simulink model "SMC_03"  (R2021a)
settings: Solver=ode14x  StartTime=0.0  StopTime=100  FixedStep=0.01  RelTol=1e-3
libraries: simulink x2
settings Model: Creator=TMP  LastModifiedBy=TMP
settings DataIOCC: SaveTime=off  ReturnWorkspaceOutputs=off

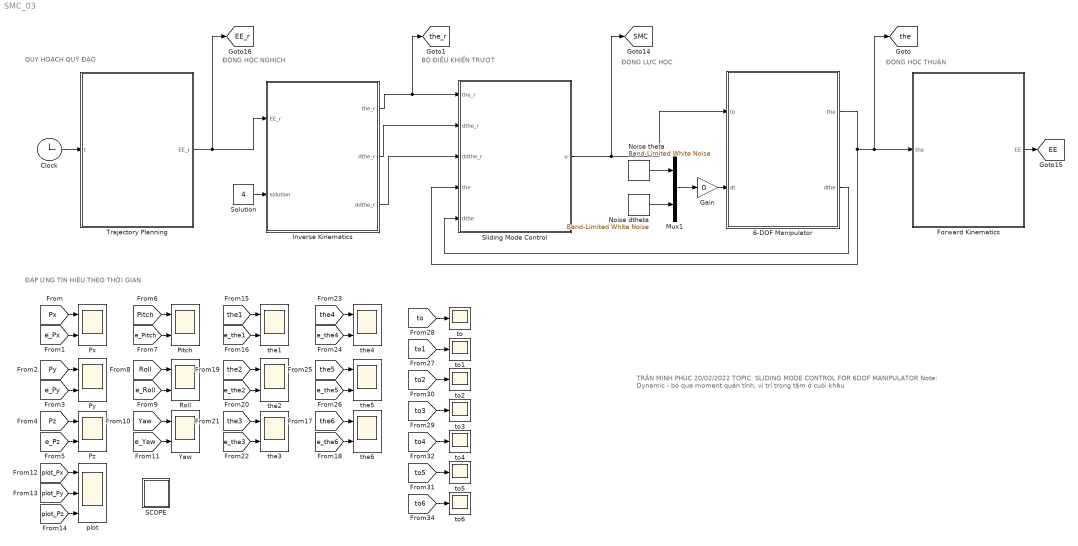
== system SMC_03 ==
  note: ĐÁP ỨNG TÍN HIÊU THEO THỜI GIAN
  note: QUY HOẠCH QUỸ ĐẠO
  note: BỘ ĐIỀU KHIỂN TRƯỢT
  note: ĐỘNG HỌC NGHỊCH
  note: ĐỌNG LỰC HỌC
  note: ĐỘNG HỌC THUẬN
  note: TRẦN MINH PHÚC
      | 20/02/2022
      | TOPIC: SLIDING MODE CONTROL FOR 6DOF MANIPULATOR
      | Note: Dynamic - bỏ qua moment quán tính, vị trí trọng tâm ở cuối khâu
  6-DOF Manipulator : Subsystem
  Clock : Clock
  Forward Kinematics : MATLAB Function  TreatAsAtomicUnit=on
  Gain : Gain  Gain=0
  Inverse Kinematics : Subsystem
  Mux1 : Mux  Inputs=2
  Noise dtheta : simulink/Sources/Band-Limited White Noise  Cov=[0.03]  Ts=0.01  seed=[23341]
  Noise theta : simulink/Sources/Band-Limited White Noise  Cov=[0.003]  Ts=0.01  seed=[23341]
  Pitch : Scope  NumInputPorts=2
  Px : Scope  NumInputPorts=2
  Py : Scope  NumInputPorts=2
  Pz : Scope  NumInputPorts=2
  Roll : Scope  NumInputPorts=2
  SCOPE : Subsystem
  Sliding Mode Control : MATLAB Function  TreatAsAtomicUnit=on
  Solution : Constant  Value=4
  Trajectory Planning : MATLAB Function  TreatAsAtomicUnit=on
  Yaw : Scope  NumInputPorts=2
  plot : Scope  NumInputPorts=3
  the{1..6} (6 alike) : Scope  NumInputPorts=2
  to{,1..6} (7 alike) : Scope
  tag scope: EE=global, EE_r=global, SMC=global, the=global, the_r=global
  wires:
  Noise theta/1 -> Mux1/1
  Noise dtheta/1 -> Mux1/2
  Mux1/1 -> Gain/1
  Clock/1 -> Trajectory Planning/1(t)
  Solution/1 -> Inverse Kinematics/2(solution)
  Trajectory Planning/1(EE_r) -> Inverse Kinematics/1(EE_r), [EE_r]
  [Px] -> Px/1
  [e_Px] -> Px/2
  [Py] -> Py/1
  [e_Py] -> Py/2
  [e_Pz] -> Pz/2
  [Pz] -> Pz/1
  [e_Yaw] -> Yaw/2
  [e_Roll] -> Roll/2
  [e_Pitch] -> Pitch/2
  [Yaw] -> Yaw/1
  [Roll] -> Roll/1
  [Pitch] -> Pitch/1
  [plot_Px] -> plot/1
  [plot_Py] -> plot/2
  [plot_Pz] -> plot/3
  [e_the5] -> the5/2
  [the5] -> the5/1
  [e_the4] -> the4/2
  [the4] -> the4/1
  [the3] -> the3/1
  [the2] -> the2/1
  [e_the6] -> the6/2
  [e_the2] -> the2/2
  [e_the1] -> the1/2
  [the6] -> the6/1
  [e_the3] -> the3/2
  [the1] -> the1/1
  [to1] -> to1/1
  [to] -> to/1
  [to6] -> to6/1
  [to5] -> to5/1
  [to4] -> to4/1
  [to3] -> to3/1
  [to2] -> to2/1
  Gain/1 -> 6-DOF Manipulator/2(dt)
  Sliding Mode Control/1(u) -> 6-DOF Manipulator/1(to), [SMC]
  6-DOF Manipulator/2(dthe) -> Sliding Mode Control/5(dthe)
  6-DOF Manipulator/1(the) -> Forward Kinematics/1(the), [the], Sliding Mode Control/4(the)
  Forward Kinematics/1(EE) -> [EE]
  Inverse Kinematics/1(the_r) -> [the_r], Sliding Mode Control/1(the_r)
  Inverse Kinematics/2(dthe_r) -> Sliding Mode Control/2(dthe_r)
  Inverse Kinematics/3(ddthe_r) -> Sliding Mode Control/3(ddthe_r)

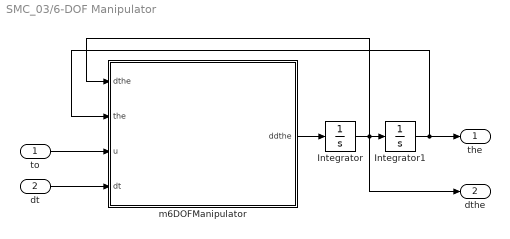
== system SMC_03/6-DOF Manipulator ==
  to : Inport
  dt : Inport  Port=2
  Integrator : Integrator  InitialCondition=[0.01;0.01;0.01;0.01;0.01;0.01]
  Integrator1 : Integrator  InitialCondition=[0.01;0.01;0.01;0.01;0.01;0.01]
  m6DOFManipulator : MATLAB Function  TreatAsAtomicUnit=on
  the : Outport
  dthe : Outport  Port=2
  wires:
  Integrator1/1 -> the/1, m6DOFManipulator/2(the)
  m6DOFManipulator/1(ddthe) -> Integrator/1
  Integrator/1 -> dthe/1, m6DOFManipulator/1(dthe), Integrator1/1
  dt/1 -> m6DOFManipulator/4(dt)
  to/1 -> m6DOFManipulator/3(u)

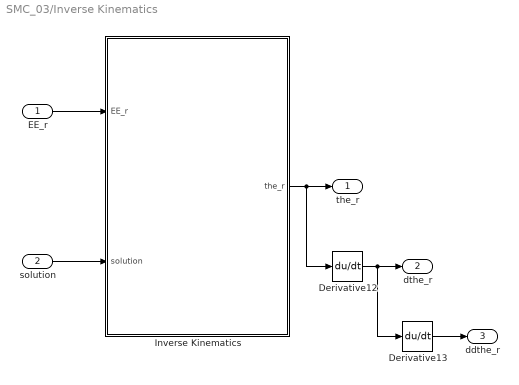
== system SMC_03/Inverse Kinematics ==
  EE_r : Inport
  solution : Inport  Port=2
  Derivative12 : Derivative
  Derivative13 : Derivative
  Inverse Kinematics : MATLAB Function  TreatAsAtomicUnit=on
  the_r : Outport  VectorParamsAs1DForOutWhenUnconnected=off
  dthe_r : Outport  Port=2  VectorParamsAs1DForOutWhenUnconnected=off
  ddthe_r : Outport  Port=3  VectorParamsAs1DForOutWhenUnconnected=off
  wires:
  EE_r/1 -> Inverse Kinematics/1(EE_r)
  solution/1 -> Inverse Kinematics/2(solution)
  Inverse Kinematics/1(the_r) -> Derivative12/1, the_r/1
  Derivative12/1 -> Derivative13/1, dthe_r/1
  Derivative13/1 -> ddthe_r/1

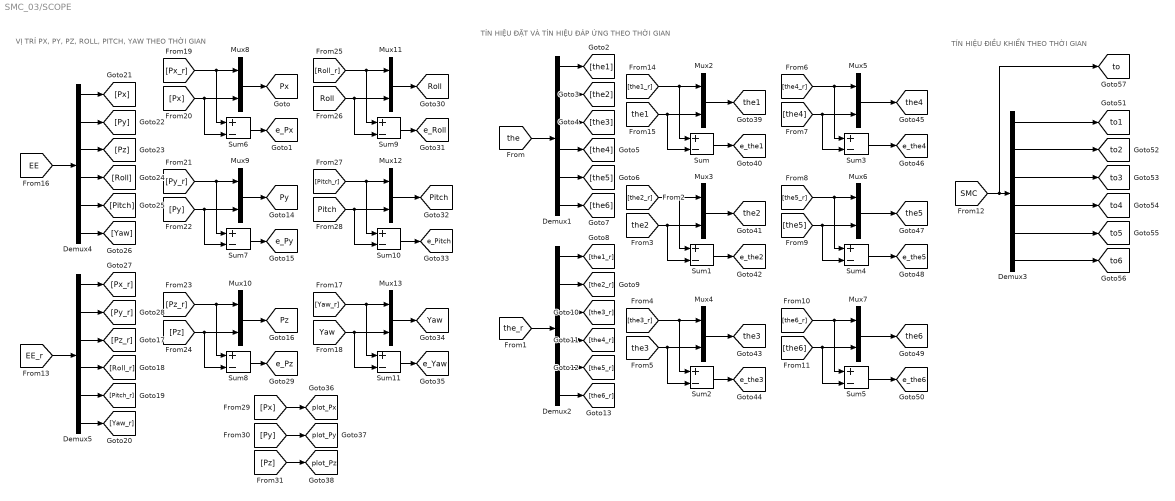
== system SMC_03/SCOPE ==
  note: TÍN HIỆU ĐIỀU KHIỂN THEO THỜI GIAN
  note: TÍN HIỆU ĐẶT VÀ TÍN HIỆU ĐÁP ỨNG THEO THỜI GIAN
  note: VỊ TRÍ PX, PY, PZ, ROLL, PITCH, YAW THEO THỜI GIAN
  Demux{1..5} (5 alike) : Demux  Outputs=6
  Mux{2..13} (12 alike) : Mux  Inputs=2
  Sum{,1..11} (12 alike) : Sum  Inputs=+-
  tag scope: Pitch=global, Px=global, Py=global, Pz=global, Roll=global, Yaw=global, e_Pitch=global, e_Px=global, e_Py=global, e_Pz=global, e_Roll=global, e_Yaw=global, e_the1=global, e_the2=global, e_the3=global, e_the4=global, e_the5=global, e_the6=global, plot_Px=global, plot_Py=global, plot_Pz=global, the1=global, the2=global, the3=global, the4=global, the5=global, the6=global, to1=global, to2=global, to3=global, to4=global, to5=global, to6=global, to=global
  wires:
  [the6] -> Sum5/2, Mux7/2
  Mux9/1 -> [Py]
  [the3] -> Sum2/2, Mux4/2
  Demux1/6 -> [the6]
  Demux5/1 -> [Px_r]
  [the1] -> Sum/2, Mux2/2
  [Py] -> Sum7/2, Mux9/2
  Demux2/2 -> [the2_r]
  Demux5/6 -> [Yaw_r]
  Demux4/4 -> [Roll]
  [Pz_r] -> Sum8/1, Mux10/1
  [the5] -> Sum4/2, Mux6/2
  [EE] -> Demux4/1
  Mux11/1 -> [Roll]
  [EE_r] -> Demux5/1
  Demux4/2 -> [Py]
  [Px_r] -> Sum6/1, Mux8/1
  Mux5/1 -> [the4]
  Demux1/4 -> [the4]
  [Pitch] -> Sum10/2, Mux12/2
  [the6_r] -> Sum5/1, Mux7/1
  Mux2/1 -> [the1]
  [the4_r] -> Sum3/1, Mux5/1
  Demux2/1 -> [the1_r]
  Demux5/5 -> [Pitch_r]
  [the1_r] -> Sum/1, Mux2/1
  Sum7/1 -> [e_Py]
  Demux4/3 -> [Pz]
  [Py_r] -> Sum7/1, Mux9/1
  Demux1/3 -> [the3]
  Demux5/2 -> [Py_r]
  Demux3/1 -> [to1]
  Demux4/6 -> [Yaw]
  [Pz] -> [plot_Pz]
  [Roll] -> Sum9/2, Mux11/2
  Demux5/3 -> [Pz_r]
  [Roll_r] -> Sum9/1, Mux11/1
  Demux2/5 -> [the5_r]
  [Px] -> Sum6/2, Mux8/2
  [the5_r] -> Sum4/1, Mux6/1
  Demux5/4 -> [Roll_r]
  [the] -> Demux1/1
  Demux1/2 -> [the2]
  Demux1/1 -> [the1]
  Mux7/1 -> [the6]
  Demux2/4 -> [the4_r]
  [Yaw_r] -> Sum11/1, Mux13/1
  [the_r] -> Demux2/1
  Demux3/3 -> [to3]
  [the2_r] -> Sum1/1, Mux3/1
  Demux4/1 -> [Px]
  [Pitch_r] -> Sum10/1, Mux12/1
  [Pz] -> Sum8/2, Mux10/2
  Demux2/6 -> [the6_r]
  [SMC] -> [to], Demux3/1
  Sum9/1 -> [e_Roll]
  [the3_r] -> Sum2/1, Mux4/1
  [Yaw] -> Sum11/2, Mux13/2
  Sum8/1 -> [e_Pz]
  Demux2/3 -> [the3_r]
  Demux1/5 -> [the5]
  [the4] -> Sum3/2, Mux5/2
  [the2] -> Sum1/2, Mux3/2
  Demux4/5 -> [Pitch]
  Sum11/1 -> [e_Yaw]
  [Px] -> [plot_Px]
  Sum6/1 -> [e_Px]
  [Py] -> [plot_Py]
  Mux3/1 -> [the2]
  Sum/1 -> [e_the1]
  Sum5/1 -> [e_the6]
  Sum2/1 -> [e_the3]
  Sum4/1 -> [e_the5]
  Mux4/1 -> [the3]
  Sum1/1 -> [e_the2]
  Demux3/4 -> [to4]
  Mux6/1 -> [the5]
  Demux3/5 -> [to5]
  Mux13/1 -> [Yaw]
  Sum3/1 -> [e_the4]
  Demux3/6 -> [to6]
  Mux10/1 -> [Pz]
  Mux8/1 -> [Px]
  Demux3/2 -> [to2]
  Mux12/1 -> [Pitch]
  Sum10/1 -> [e_Pitch]

== matlab function SMC_03/Sliding Mode Control ==
  data: the_r input; dthe_r input; ddthe_r input; the input; u output; dthe input
function u = SMC(the_r,dthe_r,ddthe_r,the,dthe)
%% Declare manipulator dynamics:
m1=0.1; m2=0.1; m3=0.1; m4=0.1; m5=0.1; m6=0.1;
I1=0; I2=0; I3=0; I4=0; I5=0; I6=1;
a1=0.75; a2=2.70; a3=0.90; d1=3.35; d4=2.95; d7=0.80;
g=9.81;
%%
e1 = the(1); e2 = the(2); e3 = the(3);
e4 = the(4); e5 = the(5); e6 = the(6);
de1 = dthe(1); de2 = dthe(2); de3 = dthe(3);
de4 = dthe(4); de5 = dthe(5); de6 = dthe(6);
%% M
M = [I1 + I2 + I3 + I4 + I5 + I6 + a1^2*m2 + a1^2*m3 + a1^2*m4 + (a2^2*m3)/2 + a1^2*m5 + (a2^2*m4)/2 + a1^2*m6 + (a2^2*m5)/2 + (a3^2*m4)/2 + (a2^2*m6)/2 + (a3^2*m5)/2 + (a3^2*m6)/2 + (d4^2*m4)/2 + (d4^2*m5)/2 + (d4^2*m6)/2 - (a2^2*m3*cos(2*e2))/2 - (a2^2*m4*cos(2*e2))/2 - (a2^2*m5*cos(2*e2))/2 - (a2^2*m6*cos(2*e2))/2 - (a3^2*m4*cos(2*e2 + 2*e3))/2 - (a3^2*m5*cos(2*e2 + 2*e3))/2 - (a3^2*m6*cos(2*e2 + 2*e3))/2 + (d4^2*m4*cos(2*e2 + 2*e3))/2 + (d4^2*m5*cos(2*e2 + 2*e3))/2 + (d4^2*m6*cos(2*e2 + 2*e3))/2 + 2*a1*d4*m4*cos(e2 + e3) + 2*a1*d4*m5*cos(e2 + e3) + 2*a1*d4*m6*cos(e2 + e3) + 2*a1*a3*m4*sin(e2 + e3) + 2*a1*a3*m5*sin(e2 + e3) + 2*a1*a3*m6*sin(e2 + e3) + a2*a3*m4*cos(e3) + a2*a3*m5*cos(e3) + a2*a3*m6*cos(e3) + 2*a1*a2*m3*sin(e2) + 2*a1*a2*m4*sin(e2) + 2*a1*a2*m5*sin(e2) + 2*a1*a2*m6*sin(e2) - a2*d4*m4*sin(e3) - a2*d4*m5*sin(e3) - a2*d4*m6*sin(e3) - a2*a3*m4*cos(2*e2 + e3) - a2*a3*m5*cos(2*e2 + e3) - a2*a3*m6*cos(2*e2 + e3) + a2*d4*m4*sin(2*e2 + e3) + a2*d4*m5*sin(2*e2 + e3) + a2*d4*m6*sin(2*e2 + e3) + a3*d4*m4*sin(2*e2 + 2*e3) + a3*d4*m5*sin(2*e2 + 2*e3) + a3*d4*m6*sin(2*e2 + 2*e3),0,0,-sin(e2 + e3)*(I4 + I5 + I6),cos(e2 + e3)*sin(e4)*(I5 + I6),I6*cos(e4)*sin(e2)*sin(e3)*sin(e5) - I6*cos(e3)*cos(e5)*sin(e2) - I6*cos(e2)*cos(e3)*cos(e4)*sin(e5) - I6*cos(e2)*cos(e5)*sin(e3);
     0,I2 + I3 + I4 + I5 + I6 + a2^2*m3 + a2^2*m4 + a2^2*m5 + a3^2*m4 + a2^2*m6 + a3^2*m5 + a3^2*m6 + d4^2*m4 + d4^2*m5 + d4^2*m6 + 2*a2*a3*m4*cos(e3) + 2*a2*a3*m5*cos(e3) + 2*a2*a3*m6*cos(e3) - 2*a2*d4*m4*sin(e3) - 2*a2*d4*m5*sin(e3) - 2*a2*d4*m6*sin(e3),I3 + I4 + I5 + I6 + a3^2*m4 + a3^2*m5 + a3^2*m6 + d4^2*m4 + d4^2*m5 + d4^2*m6 + a2*a3*m4*cos(e3) + a2*a3*m5*cos(e3) + a2*a3*m6*cos(e3) - a2*d4*m4*sin(e3) - a2*d4*m5*sin(e3) - a2*d4*m6*sin(e3),0,cos(e4)*(I5 + I6),I6*sin(e4)*sin(e5);
     0,I3 + I4 + I5 + I6 + a3^2*m4 + a3^2*m5 + a3^2*m6 + d4^2*m4 + d4^2*m5 + d4^2*m6 + a2*a3*m4*cos(e3) + a2*a3*m5*cos(e3) + a2*a3*m6*cos(e3) - a2*d4*m4*sin(e3) - a2*d4*m5*sin(e3) - a2*d4*m6*sin(e3),I3 + I4 + I5 + I6 + a3^2*m4 + a3^2*m5 + a3^2*m6 + d4^2*m4 + d4^2*m5 + d4^2*m6,0,cos(e4)*(I5 + I6),I6*sin(e4)*sin(e5);
    -sin(e2 + e3)*(I4 + I5 + I6),0,0,I4 + I5 + I6,0,I6*cos(e5);
    cos(e2 + e3)*sin(e4)*(I5 + I6),cos(e4)*(I5 + I6),cos(e4)*(I5 + I6),0,I5 + I6,0;
    I6*cos(e4)*sin(e2)*sin(e3)*sin(e5) - I6*cos(e3)*cos(e5)*sin(e2) - I6*cos(e2)*cos(e3)*cos(e4)*sin(e5) - I6*cos(e2)*cos(e5)*sin(e3),I6*sin(e4)*sin(e5),I6*sin(e4)*sin(e5),I6*cos(e5),0,I6];
%% C
C = ...
[de2*(a2^2*m3*sin(2*e2) + a2^2*m4*sin(2*e2) + a2^2*m5*sin(2*e2) + a2^2*m6*sin(2*e2) + a3^2*m4*sin(2*e2 + 2*e3) + a3^2*m5*sin(2*e2 + 2*e3) + a3^2*m6*sin(2*e2 + 2*e3) - d4^2*m4*sin(2*e2 + 2*e3) - d4^2*m5*sin(2*e2 + 2*e3) - d4^2*m6*sin(2*e2 + 2*e3) + 2*a1*a3*m4*cos(e2 + e3) + 2*a1*a3*m5*cos(e2 + e3) + 2*a1*a3*m6*cos(e2 + e3) - 2*a1*d4*m4*sin(e2 + e3) - 2*a1*d4*m5*sin(e2 + e3) - 2*a1*d4*m6*sin(e2 + e3) + 2*a1*a2*m3*cos(e2) + 2*a1*a2*m4*cos(e2) + 2*a1*a2*m5*cos(e2) + 2*a1*a2*m6*cos(e2) + 2*a2*d4*m4*cos(2*e2 + e3) + 2*a2*d4*m5*cos(2*e2 + e3) + 2*a2*d4*m6*cos(2*e2 + e3) + 2*a2*a3*m4*sin(2*e2 + e3) + 2*a2*a3*m5*sin(2*e2 + e3) + 2*a2*a3*m6*sin(2*e2 + e3) + 2*a3*d4*m4*cos(2*e2 + 2*e3) + 2*a3*d4*m5*cos(2*e2 + 2*e3) + 2*a3*d4*m6*cos(2*e2 + 2*e3)) + de3*(m4 + m5 + m6)*(a3^2*sin(2*e2 + 2*e3) - d4^2*sin(2*e2 + 2*e3) + a2*d4*cos(2*e2 + e3) + a2*a3*sin(2*e2 + e3) + 2*a3*d4*cos(2*e2 + 2*e3) + 2*a1*a3*cos(e2 + e3) - 2*a1*d4*sin(e2 + e3) - a2*d4*cos(e3) - a2*a3*sin(e3)),0,0,-cos(e2 + e3)*(de2 + de3)*(I4 + I5 + I6),-(I5 + I6)*(de2*sin(e2 + e3)*sin(e4) - de4*cos(e2 + e3)*cos(e4) + de3*sin(e2 + e3)*sin(e4)),I6*de2*(cos(e5)*sin(e2)*sin(e3) - cos(e2)*cos(e3)*cos(e5) + cos(e2)*cos(e4)*sin(e3)*sin(e5) + cos(e3)*cos(e4)*sin(e2)*sin(e5)) + I6*de3*(cos(e5)*sin(e2)*sin(e3) - cos(e2)*cos(e3)*cos(e5) + cos(e2)*cos(e4)*sin(e3)*sin(e5) + cos(e3)*cos(e4)*sin(e2)*sin(e5)) + I6*de5*(cos(e2)*sin(e3)*sin(e5) + cos(e3)*sin(e2)*sin(e5) - cos(e2)*cos(e3)*cos(e4)*cos(e5) + cos(e4)*cos(e5)*sin(e2)*sin(e3)) + I6*de4*cos(e2 + e3)*sin(e4)*sin(e5);
 (I4*de4*cos(e2 + e3))/2 + (I5*de4*cos(e2 + e3))/2 + (I6*de4*cos(e2 + e3))/2 - (a2^2*de1*m3*sin(2*e2))/2 - (a2^2*de1*m4*sin(2*e2))/2 - (a2^2*de1*m5*sin(2*e2))/2 - (a2^2*de1*m6*sin(2*e2))/2 - (a3^2*de1*m4*sin(2*e2 + 2*e3))/2 - (a3^2*de1*m5*sin(2*e2 + 2*e3))/2 - (a3^2*de1*m6*sin(2*e2 + 2*e3))/2 + (d4^2*de1*m4*sin(2*e2 + 2*e3))/2 + (d4^2*de1*m5*sin(2*e2 + 2*e3))/2 + (d4^2*de1*m6*sin(2*e2 + 2*e3))/2 + (I5*de5*sin(e2 + e3)*sin(e4))/2 + (I6*de5*sin(e2 + e3)*sin(e4))/2 - a3*d4*de1*m4*cos(2*e2 + 2*e3) - a3*d4*de1*m5*cos(2*e2 + 2*e3) - a3*d4*de1*m6*cos(2*e2 + 2*e3) + (I6*de6*cos(e2)*cos(e3)*cos(e5))/2 - a1*a3*de1*m4*cos(e2 + e3) - a1*a3*de1*m5*cos(e2 + e3) - a1*a3*de1*m6*cos(e2 + e3) - (I6*de6*cos(e5)*sin(e2)*sin(e3))/2 + a1*d4*de1*m4*sin(e2 + e3) + a1*d4*de1*m5*sin(e2 + e3) + a1*d4*de1*m6*sin(e2 + e3) - a1*a2*de1*m3*cos(e2) - a1*a2*de1*m4*cos(e2) - a1*a2*de1*m5*cos(e2) - a1*a2*de1*m6*cos(e2) - a2*d4*de1*m4*cos(2*e2 + e3) - a2*d4*de1*m5*cos(2*e2 + e3) - a2*d4*de1*m6*cos(2*e2 + e3) - a2*a3*de1*m4*sin(2*e2 + e3) - a2*a3*de1*m5*sin(2*e2 + e3) - a2*a3*de1*m6*sin(2*e2 + e3) - (I6*de6*cos(e2)*cos(e4)*sin(e3)*sin(e5))/2 - (I6*de6*cos(e3)*cos(e4)*sin(e2)*sin(e5))/2,-2*a2*de3*(d4*cos(e3) + a3*sin(e3))*(m4 + m5 + m6),-a2*de3*(d4*cos(e3) + a3*sin(e3))*(m4 + m5 + m6),(de1*cos(e2 + e3)*(I4 + I5 + I6))/2,-(sin(e4)*(2*de4 - de1*sin(e2 + e3))*(I5 + I6))/2,(I6*(2*de4*cos(e4)*sin(e5) + 2*de5*cos(e5)*sin(e4) + de1*cos(e2)*cos(e3)*cos(e5) - de1*cos(e5)*sin(e2)*sin(e3) - de1*cos(e2)*cos(e4)*sin(e3)*sin(e5) - de1*cos(e3)*cos(e4)*sin(e2)*sin(e5)))/2;
 (de4*cos(e2 + e3)*(I4 + I5 + I6))/2 - (I6*de6*(cos(e5)*sin(e2)*sin(e3) - cos(e2)*cos(e3)*cos(e5) + cos(e2)*cos(e4)*sin(e3)*sin(e5) + cos(e3)*cos(e4)*sin(e2)*sin(e5)))/2 - (de1*(m4 + m5 + m6)*(a3^2*sin(2*e2 + 2*e3) - d4^2*sin(2*e2 + 2*e3) + a2*d4*cos(2*e2 + e3) + a2*a3*sin(2*e2 + e3) + 2*a3*d4*cos(2*e2 + 2*e3) + 2*a1*a3*cos(e2 + e3) - 2*a1*d4*sin(e2 + e3) - a2*d4*cos(e3) - a2*a3*sin(e3)))/2 + (de5*sin(e2 + e3)*sin(e4)*(I5 + I6))/2,(a2*(d4*cos(e3) + a3*sin(e3))*(2*de2 - de3)*(m4 + m5 + m6))/2,(a2*de2*(d4*cos(e3) + a3*sin(e3))*(m4 + m5 + m6))/2,(de1*cos(e2 + e3)*(I4 + I5 + I6))/2,-(sin(e4)*(2*de4 - de1*sin(e2 + e3))*(I5 + I6))/2,(I6*(2*de4*cos(e4)*sin(e5) + 2*de5*cos(e5)*sin(e4) + de1*cos(e2)*cos(e3)*cos(e5) - de1*cos(e5)*sin(e2)*sin(e3) - de1*cos(e2)*cos(e4)*sin(e3)*sin(e5) - de1*cos(e3)*cos(e4)*sin(e2)*sin(e5)))/2;
 - cos(e2 + e3)*(de2 + de3)*(I4 + I5 + I6) - (de5*cos(e2 + e3)*cos(e4)*(I5 + I6))/2 - (I6*de6*cos(e2 + e3)*sin(e4)*sin(e5))/2,(de5*sin(e4)*(I5 + I6))/2 - (I6*de6*cos(e4)*sin(e5))/2,(de5*sin(e4)*(I5 + I6))/2 - (I6*de6*cos(e4)*sin(e5))/2,0,((I5 + I6)*(de2*sin(e4) + de3*sin(e4) - de1*cos(e2 + e3)*cos(e4)))/2,-(I6*sin(e5)*(2*de5 + de2*cos(e4) + de3*cos(e4) + de1*cos(e2 + e3)*sin(e4)))/2;
 - (I5 + I6)*(de2*sin(e2 + e3)*sin(e4) - de4*cos(e2 + e3)*cos(e4) + de3*sin(e2 + e3)*sin(e4)) - (I6*de6*(cos(e2)*sin(e3)*sin(e5) + cos(e3)*sin(e2)*sin(e5) - cos(e2)*cos(e3)*cos(e4)*cos(e5) + cos(e4)*cos(e5)*sin(e2)*sin(e3)))/2,- de4*sin(e4)*(I5 + I6) - (I6*de6*cos(e5)*sin(e4))/2,- de4*sin(e4)*(I5 + I6) - (I6*de6*cos(e5)*sin(e4))/2,(I6*de6*sin(e5))/2,0,-(I6*(de2*cos(e5)*sin(e4) - de4*sin(e5) + de3*cos(e5)*sin(e4) + de1*cos(e2)*sin(e3)*sin(e5) + de1*cos(e3)*sin(e2)*sin(e5) + de1*cos(e4)*cos(e5)*sin(e2)*sin(e3) - de1*cos(e2)*cos(e3)*cos(e4)*cos(e5)))/2;
 I6*de2*(cos(e5)*sin(e2)*sin(e3) - cos(e2)*cos(e3)*cos(e5) + cos(e2)*cos(e4)*sin(e3)*sin(e5) + cos(e3)*cos(e4)*sin(e2)*sin(e5)) + I6*de3*(cos(e5)*sin(e2)*sin(e3) - cos(e2)*cos(e3)*cos(e5) + cos(e2)*cos(e4)*sin(e3)*sin(e5) + cos(e3)*cos(e4)*sin(e2)*sin(e5)) + I6*de5*(cos(e2)*sin(e3)*sin(e5) + cos(e3)*sin(e2)*sin(e5) - cos(e2)*cos(e3)*cos(e4)*cos(e5) + cos(e4)*cos(e5)*sin(e2)*sin(e3)) + I6*de4*cos(e2 + e3)*sin(e4)*sin(e5),I6*de4*cos(e4)*sin(e5) + I6*de5*cos(e5)*sin(e4),I6*de4*cos(e4)*sin(e5) + I6*de5*cos(e5)*sin(e4),-I6*de5*sin(e5),0,0];
%% V
V = C*dthe;
%% G
G = ...
[    
                                                                                                                                                                                              0;
g*(a2*m3*sin(e2) + a2*m4*sin(e2) + a2*m5*sin(e2) + a2*m6*sin(e2) + d4*m4*cos(e2 + e3) + d4*m5*cos(e2 + e3) + d4*m6*cos(e2 + e3) + a3*m4*sin(e2 + e3) + a3*m5*sin(e2 + e3) + a3*m6*sin(e2 + e3));
                                                                                                                                           g*(d4*cos(e2 + e3) + a3*sin(e2 + e3))*(m4 + m5 + m6);
                                                                                                                                                                                              0;
                                                                                                                                                                                              0;
                                                                                                                                                                                              0];

%% Control:
% Controler parameters
% % with noise
% lamda = 50;
% K = 30;
% K1 = 50;

% without noise
lamda = diag([20,20,20,20,20,20]);
K = diag([20,20,20,20,20,20]);
K1 = diag([5,5,5,5,5,5]);

% Designed sliding mode control
f_x = -inv(M)*V - inv(M)*G;
g_x = inv(M);
e1 = the - the_r;
e2 = dthe - dthe_r;
s = lamda*e1 + e2;
u = inv(g_x)*(-f_x + ddthe_r - lamda*e2 - K1*s - K*sign(s));
% sat
% u = inv(g_x)*(-f_x + ddthe_r - lamda*e2 - K1*s - K*min(0.1, max(-0.1, s)));

== matlab function SMC_03/6-DOF Manipulator/m6DOFManipulator ==
  data: dthe input; the input; u input; ddthe output; dt input
function ddthe  = m6DOFManipulator(dthe,the,u,dt)
%% Declare:
m1=0.1; m2=0.1; m3=0.1; m4=0.1; m5=0.1; m6=0.1;
I1=0; I2=0; I3=0; I4=0; I5=0; I6=1;
a1=0.75; a2=2.70; a3=0.90; d1=3.35; d4=2.95; d7=0.80;
g=9.81;
%%
e1 = the(1) + dt(1); e2 = the(2) + dt(1); e3 = the(3) + dt(1);
e4 = the(4) + dt(1); e5 = the(5) + dt(1); e6 = the(6) + dt(1);
de1 = dthe(1) + dt(2); de2 = dthe(2) + dt(2); de3 = dthe(3) + dt(2);
de4 = dthe(4) + dt(2); de5 = dthe(5) + dt(2); de6 = dthe(6) + dt(2);
%% M
M = [I1 + I2 + I3 + I4 + I5 + I6 + a1^2*m2 + a1^2*m3 + a1^2*m4 + (a2^2*m3)/2 + a1^2*m5 + (a2^2*m4)/2 + a1^2*m6 + (a2^2*m5)/2 + (a3^2*m4)/2 + (a2^2*m6)/2 + (a3^2*m5)/2 + (a3^2*m6)/2 + (d4^2*m4)/2 + (d4^2*m5)/2 + (d4^2*m6)/2 - (a2^2*m3*cos(2*e2))/2 - (a2^2*m4*cos(2*e2))/2 - (a2^2*m5*cos(2*e2))/2 - (a2^2*m6*cos(2*e2))/2 - (a3^2*m4*cos(2*e2 + 2*e3))/2 - (a3^2*m5*cos(2*e2 + 2*e3))/2 - (a3^2*m6*cos(2*e2 + 2*e3))/2 + (d4^2*m4*cos(2*e2 + 2*e3))/2 + (d4^2*m5*cos(2*e2 + 2*e3))/2 + (d4^2*m6*cos(2*e2 + 2*e3))/2 + 2*a1*d4*m4*cos(e2 + e3) + 2*a1*d4*m5*cos(e2 + e3) + 2*a1*d4*m6*cos(e2 + e3) + 2*a1*a3*m4*sin(e2 + e3) + 2*a1*a3*m5*sin(e2 + e3) + 2*a1*a3*m6*sin(e2 + e3) + a2*a3*m4*cos(e3) + a2*a3*m5*cos(e3) + a2*a3*m6*cos(e3) + 2*a1*a2*m3*sin(e2) + 2*a1*a2*m4*sin(e2) + 2*a1*a2*m5*sin(e2) + 2*a1*a2*m6*sin(e2) - a2*d4*m4*sin(e3) - a2*d4*m5*sin(e3) - a2*d4*m6*sin(e3) - a2*a3*m4*cos(2*e2 + e3) - a2*a3*m5*cos(2*e2 + e3) - a2*a3*m6*cos(2*e2 + e3) + a2*d4*m4*sin(2*e2 + e3) + a2*d4*m5*sin(2*e2 + e3) + a2*d4*m6*sin(2*e2 + e3) + a3*d4*m4*sin(2*e2 + 2*e3) + a3*d4*m5*sin(2*e2 + 2*e3) + a3*d4*m6*sin(2*e2 + 2*e3),0,0,-sin(e2 + e3)*(I4 + I5 + I6),cos(e2 + e3)*sin(e4)*(I5 + I6),I6*cos(e4)*sin(e2)*sin(e3)*sin(e5) - I6*cos(e3)*cos(e5)*sin(e2) - I6*cos(e2)*cos(e3)*cos(e4)*sin(e5) - I6*cos(e2)*cos(e5)*sin(e3);
     0,I2 + I3 + I4 + I5 + I6 + a2^2*m3 + a2^2*m4 + a2^2*m5 + a3^2*m4 + a2^2*m6 + a3^2*m5 + a3^2*m6 + d4^2*m4 + d4^2*m5 + d4^2*m6 + 2*a2*a3*m4*cos(e3) + 2*a2*a3*m5*cos(e3) + 2*a2*a3*m6*cos(e3) - 2*a2*d4*m4*sin(e3) - 2*a2*d4*m5*sin(e3) - 2*a2*d4*m6*sin(e3),I3 + I4 + I5 + I6 + a3^2*m4 + a3^2*m5 + a3^2*m6 + d4^2*m4 + d4^2*m5 + d4^2*m6 + a2*a3*m4*cos(e3) + a2*a3*m5*cos(e3) + a2*a3*m6*cos(e3) - a2*d4*m4*sin(e3) - a2*d4*m5*sin(e3) - a2*d4*m6*sin(e3),0,cos(e4)*(I5 + I6),I6*sin(e4)*sin(e5);
     0,I3 + I4 + I5 + I6 + a3^2*m4 + a3^2*m5 + a3^2*m6 + d4^2*m4 + d4^2*m5 + d4^2*m6 + a2*a3*m4*cos(e3) + a2*a3*m5*cos(e3) + a2*a3*m6*cos(e3) - a2*d4*m4*sin(e3) - a2*d4*m5*sin(e3) - a2*d4*m6*sin(e3),I3 + I4 + I5 + I6 + a3^2*m4 + a3^2*m5 + a3^2*m6 + d4^2*m4 + d4^2*m5 + d4^2*m6,0,cos(e4)*(I5 + I6),I6*sin(e4)*sin(e5);
    -sin(e2 + e3)*(I4 + I5 + I6),0,0,I4 + I5 + I6,0,I6*cos(e5);
    cos(e2 + e3)*sin(e4)*(I5 + I6),cos(e4)*(I5 + I6),cos(e4)*(I5 + I6),0,I5 + I6,0;
    I6*cos(e4)*sin(e2)*sin(e3)*sin(e5) - I6*cos(e3)*cos(e5)*sin(e2) - I6*cos(e2)*cos(e3)*cos(e4)*sin(e5) - I6*cos(e2)*cos(e5)*sin(e3),I6*sin(e4)*sin(e5),I6*sin(e4)*sin(e5),I6*cos(e5),0,I6];
%% C
C = ...
[de2*(a2^2*m3*sin(2*e2) + a2^2*m4*sin(2*e2) + a2^2*m5*sin(2*e2) + a2^2*m6*sin(2*e2) + a3^2*m4*sin(2*e2 + 2*e3) + a3^2*m5*sin(2*e2 + 2*e3) + a3^2*m6*sin(2*e2 + 2*e3) - d4^2*m4*sin(2*e2 + 2*e3) - d4^2*m5*sin(2*e2 + 2*e3) - d4^2*m6*sin(2*e2 + 2*e3) + 2*a1*a3*m4*cos(e2 + e3) + 2*a1*a3*m5*cos(e2 + e3) + 2*a1*a3*m6*cos(e2 + e3) - 2*a1*d4*m4*sin(e2 + e3) - 2*a1*d4*m5*sin(e2 + e3) - 2*a1*d4*m6*sin(e2 + e3) + 2*a1*a2*m3*cos(e2) + 2*a1*a2*m4*cos(e2) + 2*a1*a2*m5*cos(e2) + 2*a1*a2*m6*cos(e2) + 2*a2*d4*m4*cos(2*e2 + e3) + 2*a2*d4*m5*cos(2*e2 + e3) + 2*a2*d4*m6*cos(2*e2 + e3) + 2*a2*a3*m4*sin(2*e2 + e3) + 2*a2*a3*m5*sin(2*e2 + e3) + 2*a2*a3*m6*sin(2*e2 + e3) + 2*a3*d4*m4*cos(2*e2 + 2*e3) + 2*a3*d4*m5*cos(2*e2 + 2*e3) + 2*a3*d4*m6*cos(2*e2 + 2*e3)) + de3*(m4 + m5 + m6)*(a3^2*sin(2*e2 + 2*e3) - d4^2*sin(2*e2 + 2*e3) + a2*d4*cos(2*e2 + e3) + a2*a3*sin(2*e2 + e3) + 2*a3*d4*cos(2*e2 + 2*e3) + 2*a1*a3*cos(e2 + e3) - 2*a1*d4*sin(e2 + e3) - a2*d4*cos(e3) - a2*a3*sin(e3)),0,0,-cos(e2 + e3)*(de2 + de3)*(I4 + I5 + I6),-(I5 + I6)*(de2*sin(e2 + e3)*sin(e4) - de4*cos(e2 + e3)*cos(e4) + de3*sin(e2 + e3)*sin(e4)),I6*de2*(cos(e5)*sin(e2)*sin(e3) - cos(e2)*cos(e3)*cos(e5) + cos(e2)*cos(e4)*sin(e3)*sin(e5) + cos(e3)*cos(e4)*sin(e2)*sin(e5)) + I6*de3*(cos(e5)*sin(e2)*sin(e3) - cos(e2)*cos(e3)*cos(e5) + cos(e2)*cos(e4)*sin(e3)*sin(e5) + cos(e3)*cos(e4)*sin(e2)*sin(e5)) + I6*de5*(cos(e2)*sin(e3)*sin(e5) + cos(e3)*sin(e2)*sin(e5) - cos(e2)*cos(e3)*cos(e4)*cos(e5) + cos(e4)*cos(e5)*sin(e2)*sin(e3)) + I6*de4*cos(e2 + e3)*sin(e4)*sin(e5);
 (I4*de4*cos(e2 + e3))/2 + (I5*de4*cos(e2 + e3))/2 + (I6*de4*cos(e2 + e3))/2 - (a2^2*de1*m3*sin(2*e2))/2 - (a2^2*de1*m4*sin(2*e2))/2 - (a2^2*de1*m5*sin(2*e2))/2 - (a2^2*de1*m6*sin(2*e2))/2 - (a3^2*de1*m4*sin(2*e2 + 2*e3))/2 - (a3^2*de1*m5*sin(2*e2 + 2*e3))/2 - (a3^2*de1*m6*sin(2*e2 + 2*e3))/2 + (d4^2*de1*m4*sin(2*e2 + 2*e3))/2 + (d4^2*de1*m5*sin(2*e2 + 2*e3))/2 + (d4^2*de1*m6*sin(2*e2 + 2*e3))/2 + (I5*de5*sin(e2 + e3)*sin(e4))/2 + (I6*de5*sin(e2 + e3)*sin(e4))/2 - a3*d4*de1*m4*cos(2*e2 + 2*e3) - a3*d4*de1*m5*cos(2*e2 + 2*e3) - a3*d4*de1*m6*cos(2*e2 + 2*e3) + (I6*de6*cos(e2)*cos(e3)*cos(e5))/2 - a1*a3*de1*m4*cos(e2 + e3) - a1*a3*de1*m5*cos(e2 + e3) - a1*a3*de1*m6*cos(e2 + e3) - (I6*de6*cos(e5)*sin(e2)*sin(e3))/2 + a1*d4*de1*m4*sin(e2 + e3) + a1*d4*de1*m5*sin(e2 + e3) + a1*d4*de1*m6*sin(e2 + e3) - a1*a2*de1*m3*cos(e2) - a1*a2*de1*m4*cos(e2) - a1*a2*de1*m5*cos(e2) - a1*a2*de1*m6*cos(e2) - a2*d4*de1*m4*cos(2*e2 + e3) - a2*d4*de1*m5*cos(2*e2 + e3) - a2*d4*de1*m6*cos(2*e2 + e3) - a2*a3*de1*m4*sin(2*e2 + e3) - a2*a3*de1*m5*sin(2*e2 + e3) - a2*a3*de1*m6*sin(2*e2 + e3) - (I6*de6*cos(e2)*cos(e4)*sin(e3)*sin(e5))/2 - (I6*de6*cos(e3)*cos(e4)*sin(e2)*sin(e5))/2,-2*a2*de3*(d4*cos(e3) + a3*sin(e3))*(m4 + m5 + m6),-a2*de3*(d4*cos(e3) + a3*sin(e3))*(m4 + m5 + m6),(de1*cos(e2 + e3)*(I4 + I5 + I6))/2,-(sin(e4)*(2*de4 - de1*sin(e2 + e3))*(I5 + I6))/2,(I6*(2*de4*cos(e4)*sin(e5) + 2*de5*cos(e5)*sin(e4) + de1*cos(e2)*cos(e3)*cos(e5) - de1*cos(e5)*sin(e2)*sin(e3) - de1*cos(e2)*cos(e4)*sin(e3)*sin(e5) - de1*cos(e3)*cos(e4)*sin(e2)*sin(e5)))/2;
 (de4*cos(e2 + e3)*(I4 + I5 + I6))/2 - (I6*de6*(cos(e5)*sin(e2)*sin(e3) - cos(e2)*cos(e3)*cos(e5) + cos(e2)*cos(e4)*sin(e3)*sin(e5) + cos(e3)*cos(e4)*sin(e2)*sin(e5)))/2 - (de1*(m4 + m5 + m6)*(a3^2*sin(2*e2 + 2*e3) - d4^2*sin(2*e2 + 2*e3) + a2*d4*cos(2*e2 + e3) + a2*a3*sin(2*e2 + e3) + 2*a3*d4*cos(2*e2 + 2*e3) + 2*a1*a3*cos(e2 + e3) - 2*a1*d4*sin(e2 + e3) - a2*d4*cos(e3) - a2*a3*sin(e3)))/2 + (de5*sin(e2 + e3)*sin(e4)*(I5 + I6))/2,(a2*(d4*cos(e3) + a3*sin(e3))*(2*de2 - de3)*(m4 + m5 + m6))/2,(a2*de2*(d4*cos(e3) + a3*sin(e3))*(m4 + m5 + m6))/2,(de1*cos(e2 + e3)*(I4 + I5 + I6))/2,-(sin(e4)*(2*de4 - de1*sin(e2 + e3))*(I5 + I6))/2,(I6*(2*de4*cos(e4)*sin(e5) + 2*de5*cos(e5)*sin(e4) + de1*cos(e2)*cos(e3)*cos(e5) - de1*cos(e5)*sin(e2)*sin(e3) - de1*cos(e2)*cos(e4)*sin(e3)*sin(e5) - de1*cos(e3)*cos(e4)*sin(e2)*sin(e5)))/2;
 - cos(e2 + e3)*(de2 + de3)*(I4 + I5 + I6) - (de5*cos(e2 + e3)*cos(e4)*(I5 + I6))/2 - (I6*de6*cos(e2 + e3)*sin(e4)*sin(e5))/2,(de5*sin(e4)*(I5 + I6))/2 - (I6*de6*cos(e4)*sin(e5))/2,(de5*sin(e4)*(I5 + I6))/2 - (I6*de6*cos(e4)*sin(e5))/2,0,((I5 + I6)*(de2*sin(e4) + de3*sin(e4) - de1*cos(e2 + e3)*cos(e4)))/2,-(I6*sin(e5)*(2*de5 + de2*cos(e4) + de3*cos(e4) + de1*cos(e2 + e3)*sin(e4)))/2;
 - (I5 + I6)*(de2*sin(e2 + e3)*sin(e4) - de4*cos(e2 + e3)*cos(e4) + de3*sin(e2 + e3)*sin(e4)) - (I6*de6*(cos(e2)*sin(e3)*sin(e5) + cos(e3)*sin(e2)*sin(e5) - cos(e2)*cos(e3)*cos(e4)*cos(e5) + cos(e4)*cos(e5)*sin(e2)*sin(e3)))/2,- de4*sin(e4)*(I5 + I6) - (I6*de6*cos(e5)*sin(e4))/2,- de4*sin(e4)*(I5 + I6) - (I6*de6*cos(e5)*sin(e4))/2,(I6*de6*sin(e5))/2,0,-(I6*(de2*cos(e5)*sin(e4) - de4*sin(e5) + de3*cos(e5)*sin(e4) + de1*cos(e2)*sin(e3)*sin(e5) + de1*cos(e3)*sin(e2)*sin(e5) + de1*cos(e4)*cos(e5)*sin(e2)*sin(e3) - de1*cos(e2)*cos(e3)*cos(e4)*cos(e5)))/2;
 I6*de2*(cos(e5)*sin(e2)*sin(e3) - cos(e2)*cos(e3)*cos(e5) + cos(e2)*cos(e4)*sin(e3)*sin(e5) + cos(e3)*cos(e4)*sin(e2)*sin(e5)) + I6*de3*(cos(e5)*sin(e2)*sin(e3) - cos(e2)*cos(e3)*cos(e5) + cos(e2)*cos(e4)*sin(e3)*sin(e5) + cos(e3)*cos(e4)*sin(e2)*sin(e5)) + I6*de5*(cos(e2)*sin(e3)*sin(e5) + cos(e3)*sin(e2)*sin(e5) - cos(e2)*cos(e3)*cos(e4)*cos(e5) + cos(e4)*cos(e5)*sin(e2)*sin(e3)) + I6*de4*cos(e2 + e3)*sin(e4)*sin(e5),I6*de4*cos(e4)*sin(e5) + I6*de5*cos(e5)*sin(e4),I6*de4*cos(e4)*sin(e5) + I6*de5*cos(e5)*sin(e4),-I6*de5*sin(e5),0,0];
%% V
V = C*dthe;
%% G
G = ...
[    
                                                                                                                                                                                              0;
g*(a2*m3*sin(e2) + a2*m4*sin(e2) + a2*m5*sin(e2) + a2*m6*sin(e2) + d4*m4*cos(e2 + e3) + d4*m5*cos(e2 + e3) + d4*m6*cos(e2 + e3) + a3*m4*sin(e2 + e3) + a3*m5*sin(e2 + e3) + a3*m6*sin(e2 + e3));
                                                                                                                                           g*(d4*cos(e2 + e3) + a3*sin(e2 + e3))*(m4 + m5 + m6);
                                                                                                                                                                                              0;
                                                                                                                                                                                              0;
                                                                                                                                                                                              0];
%% 
ddthe=inv(M)*(u - C*dthe - G);

== matlab function SMC_03/Trajectory Planning ==
  data: t input; EE_r output
function EE_r = TrajectoryPlanning(t)
f=0.01; %hz
Px_r = 400;
Py_r = 0+50*cos(2*pi*f*t);
Pz_r = 650+50*sin(2*pi*f*t);
roll_r=0.5;
pitch_r=0.5;
yaw_r=0.5;
EE_r = [Px_r,Py_r,Pz_r,roll_r,pitch_r,yaw_r];

== matlab function SMC_03/Forward Kinematics ==
  data: the input; EE output
function EE  = FK_6DOF(the)
the1 = the(1);
the2 = the(2);
the3 = the(3);
the4 = the(4);
the5 = the(5);
the6 = the(6);
a1=75; a2=270; a3=90; d1=335; d4=295; d7=80;

T_0_EE = ...
[ cos(the6)*(cos(the5)*sin(the1)*sin(the4) + cos(the2 + the3)*cos(the1)*sin(the5) + cos(the1)*cos(the2)*cos(the4)*cos(the5)*sin(the3) + cos(the1)*cos(the3)*cos(the4)*cos(the5)*sin(the2)) - sin(the6)*(cos(the1)*cos(the2)*sin(the3)*sin(the4) - cos(the4)*sin(the1) + cos(the1)*cos(the3)*sin(the2)*sin(the4)), - cos(the6)*(cos(the1)*cos(the2)*sin(the3)*sin(the4) - cos(the4)*sin(the1) + cos(the1)*cos(the3)*sin(the2)*sin(the4)) - sin(the6)*(cos(the5)*sin(the1)*sin(the4) + cos(the2 + the3)*cos(the1)*sin(the5) + cos(the1)*cos(the2)*cos(the4)*cos(the5)*sin(the3) + cos(the1)*cos(the3)*cos(the4)*cos(the5)*sin(the2)), cos(the2 + the3)*cos(the1)*cos(the5) - sin(the5)*(sin(the1)*sin(the4) + cos(the1)*cos(the2)*cos(the4)*sin(the3) + cos(the1)*cos(the3)*cos(the4)*sin(the2)), a1*cos(the1) + a2*cos(the1)*sin(the2) + d4*cos(the1)*cos(the2)*cos(the3) + a3*cos(the1)*cos(the2)*sin(the3) + a3*cos(the1)*cos(the3)*sin(the2) - d4*cos(the1)*sin(the2)*sin(the3) - d7*sin(the1)*sin(the4)*sin(the5) + d7*cos(the1)*cos(the2)*cos(the3)*cos(the5) - d7*cos(the1)*cos(the5)*sin(the2)*sin(the3) - d7*cos(the1)*cos(the2)*cos(the4)*sin(the3)*sin(the5) - d7*cos(the1)*cos(the3)*cos(the4)*sin(the2)*sin(the5);
  cos(the6)*(cos(the2 + the3)*sin(the1)*sin(the5) - cos(the1)*cos(the5)*sin(the4) + cos(the2)*cos(the4)*cos(the5)*sin(the1)*sin(the3) + cos(the3)*cos(the4)*cos(the5)*sin(the1)*sin(the2)) - sin(the6)*(cos(the1)*cos(the4) + cos(the2)*sin(the1)*sin(the3)*sin(the4) + cos(the3)*sin(the1)*sin(the2)*sin(the4)), - cos(the6)*(cos(the1)*cos(the4) + cos(the2)*sin(the1)*sin(the3)*sin(the4) + cos(the3)*sin(the1)*sin(the2)*sin(the4)) - sin(the6)*(cos(the2 + the3)*sin(the1)*sin(the5) - cos(the1)*cos(the5)*sin(the4) + cos(the2)*cos(the4)*cos(the5)*sin(the1)*sin(the3) + cos(the3)*cos(the4)*cos(the5)*sin(the1)*sin(the2)), cos(the2 + the3)*cos(the5)*sin(the1) - sin(the5)*(cos(the2)*cos(the4)*sin(the1)*sin(the3) - cos(the1)*sin(the4) + cos(the3)*cos(the4)*sin(the1)*sin(the2)), a1*sin(the1) + a2*sin(the1)*sin(the2) + d4*cos(the2)*cos(the3)*sin(the1) + a3*cos(the2)*sin(the1)*sin(the3) + a3*cos(the3)*sin(the1)*sin(the2) + d7*cos(the1)*sin(the4)*sin(the5) - d4*sin(the1)*sin(the2)*sin(the3) + d7*cos(the2)*cos(the3)*cos(the5)*sin(the1) - d7*cos(the5)*sin(the1)*sin(the2)*sin(the3) - d7*cos(the2)*cos(the4)*sin(the1)*sin(the3)*sin(the5) - d7*cos(the3)*cos(the4)*sin(the1)*sin(the2)*sin(the5);
                                                                                                                                                                                          - cos(the6)*(sin(the2 + the3)*sin(the5) - cos(the2 + the3)*cos(the4)*cos(the5)) - cos(the2 + the3)*sin(the4)*sin(the6),                                                                                                                                                                                             sin(the6)*(sin(the2 + the3)*sin(the5) - cos(the2 + the3)*cos(the4)*cos(the5)) - cos(the2 + the3)*cos(the6)*sin(the4),                                                                                        - sin(the2 + the3)*cos(the5) - cos(the2 + the3)*cos(the4)*sin(the5),                                                                                                                                        d1 + a2*cos(the2) + a3*cos(the2)*cos(the3) - d4*cos(the2)*sin(the3) - d4*cos(the3)*sin(the2) - a3*sin(the2)*sin(the3) - d7*cos(the2)*cos(the5)*sin(the3) - d7*cos(the3)*cos(the5)*sin(the2) - d7*cos(the2)*cos(the3)*cos(the4)*sin(the5) + d7*cos(the4)*sin(the2)*sin(the3)*sin(the5);
                                                                                                                                                                                                                                                                                                               0,                                                                                                                                                                                                                                                                                                                0,                                                                                                                                                          0,                                                                                                                                                                                                                                                                                                                                                                                                                            1];
 
r11 = T_0_EE(1,1);
r21 = T_0_EE(2,1);
r31 = T_0_EE(3,1);
r12 = T_0_EE(1,2);
r22 = T_0_EE(2,2);
r32 = T_0_EE(3,2);
r13 = T_0_EE(1,3);
r23 = T_0_EE(2,3);
r33 = T_0_EE(3,3);
pitch = atan2(-r31,sqrt(r11^2+r21^2));
yaw = atan2(r21/cos(pitch),r11/cos(pitch));
roll = atan2(r32/cos(pitch),r33/cos(pitch));
Px = T_0_EE(1,4);
Py = T_0_EE(2,4);
Pz = T_0_EE(3,4);
EE = [Px,Py,Pz,roll,pitch,yaw];

== matlab function SMC_03/Inverse Kinematics/Inverse Kinematics ==
  data: EE_r input; the_r output; solution input
function the_r  = fcn(EE_r,solution)
a1=75; a2=270; a3=90; d1=335; d4=295; d7=80;
emt = zeros(8,6);
m = 0;
px = EE_r(1);
py = EE_r(2);
pz = EE_r(3);
roll = EE_r(4);
pitch = EE_r(5);
yaw =  EE_r(6);
r11 = cos(yaw)*cos(pitch);
r21 = sin(yaw)*cos(pitch);
r31 = -sin(pitch);
r12 = cos(yaw)*sin(pitch)*sin(roll) - sin(yaw)*cos(roll);
r22 = sin(yaw)*sin(pitch)*sin(roll) + cos(yaw)*cos(roll);
r32 = cos(pitch)*sin(roll);
r13 = cos(yaw)*sin(pitch)*cos(roll) + sin(yaw)*sin(roll);
r23 = sin(yaw)*sin(pitch)*cos(roll) - cos(yaw)*sin(roll);
r33 = cos(pitch)*cos(roll);
%% Inverse Kinematics
% Find the1
a_1 = py - r23*d7;
b_1 = - px + r13*d7;
d_1 = 0;
the11 = basic_01(a_1,b_1,d_1);

for i = 1:2
    % Find the2
    u = cos(the11(i))*(px-d7*r13) + sin(the11(i))*(py-r23*d7) - a1;
    v = pz - d1 - r33*d7;
    a_2 = v;
    b_2 = u;
    d_2 = (a3^2+d4^2-u^2-v^2-a2^2)/(-2*a2);
    the22 = basic_01(a_2,b_2,d_2);
    
    for j = 1:2
        % Find the3
        a_3 = a3;
        b_3 = d4;
        c_3 = u*sin(the22(j)) + v*cos(the22(j)) - a2;
        d_3 = u*cos(the22(j)) - v*sin(the22(j));
        the33 = basic_02(a_3,b_3,c_3,d_3);
        
        % Find the5
        c5 = (r13*cos(the11(i))*cos(the22(j)) - r33*sin(the22(j)) + r23*cos(the22(j))*sin(the11(i)))*cos(the33) - (r33*cos(the22(j)) + r13*cos(the11(i))*sin(the22(j)) + r23*sin(the11(i))*sin(the22(j)))*sin(the33);
        the55 = basic_01(1,0,c5);
        
        for k = 1:2
            % Find the4
            m = m+1;
            s4 = (r23*cos(the11(i)) - r13*sin(the11(i)))/(sin(the55(k)));
            c4 = (r33*cos(the22(j)) + r13*cos(the11(i))*sin(the22(j)) + r23*sin(the11(i))*sin(the22(j)) + sin(the33)*cos(the55(k))) / (-cos(the33)*sin(the55(k)));
            the44 = atan2(s4,c4);
            
            % Find the6
            a_6 = r21*cos(the11(i)) - r11*sin(the11(i));
            b_6 = r22*cos(the11(i)) - r12*sin(the11(i));
            c_6 = -sin(the44)*cos(the55(k));
            d_6 = cos(the44);
            the66 = basic_02(a_6,b_6,c_6,-d_6);
            emt(m,:)=[the11(i),the22(j),the33,the44,the55(k),the66];
        end
    end
end
% the = emt(solution,:);
the1 = emt(solution,1);
the2 = emt(solution,2);
the3 = emt(solution,3);
the4 = emt(solution,4);
the5 = emt(solution,5);
the6 = emt(solution,6);
the_r = [the1;the2;the3;the4;the5;the6];
